simulink model "SortPeriodSimulationOpenLoop"  (R2020b)
settings: Solver=VariableStepAuto  StartTime=0.0  StopTime=10.0  RelTol=1e-3
values from neighbouring files (symbols this model uses):
  AShortPeriod = AtotalLong(2:3,2:3)    [generateAutopilotSmallPeriod.m]    (also in generateAutopilotVariables.m = [-1.98701,   66.6537)
  BShortPeriod = [ -50.1873 ... (first row only)    [generateAutopilotSmallPeriod.m]    (also in generateAutopilotVariables.m = [-139.3498)
  CShortPeriod = [1,     0 ... (first row only)    [generateAutopilotSmallPeriod.m]    (also in generateAutopilotVariables.m)
  DShortPeriod = [0 ... (first row only)    [generateAutopilotSmallPeriod.m]    (also in generateAutopilotVariables.m)
settings Model: Creator=Antonis Kantounias  LastModifiedBy=Antonis Kantounias

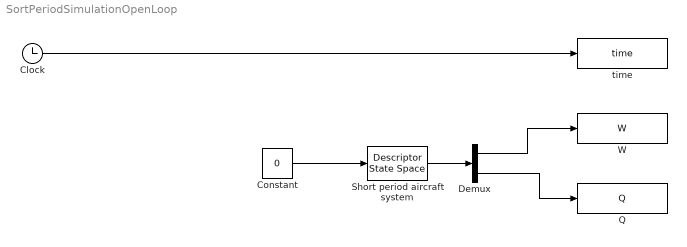
== system SortPeriodSimulationOpenLoop ==
  Clock : Clock
  Constant : Constant  Value=0
  Demux : Demux  Outputs=2
  Q : ToWorkspace  VariableName=Q  SaveFormat=Timeseries  SampleTime=-1
  Short period aircraft system : DescriptorStateSpace  E=EShordPeriod  A=AShortPeriod  B=BShortPeriod  C=CShortPeriod  D=DShortPeriod  InitialCondition=[0,1]
  W : ToWorkspace  VariableName=W  SaveFormat=Timeseries  SampleTime=-1
  time : ToWorkspace  VariableName=time  SaveFormat=Timeseries  SampleTime=-1
  wires:
  Clock/1 -> time/1
  Demux/2 -> Q/1
  Constant/1 -> Short period aircraft system/1
  Short period aircraft system/1 -> Demux/1
  Demux/1 -> W/1
